simulink model "ref_submodel2"  (R2022b)
settings: Solver=FixedStepDiscrete  StartTime=0.0  StopTime=inf  RelTol=1e-3  EnableMultiTasking=on
libraries: speedgoatlib_IO135 x2, simulink x2, hdlsllib x2, slrealtimeloglib x1
settings Model: Creator=dmankov  LastModifiedBy=padlewsk
settings SolverCC: ConcurrentTasks=on  AlgebraicLoopSolver=TrustRegion  PositivePriorityOrder=on  AutoInsertRateTranBlk=on  InsertRTBMode=Never (minimum delay)
settings DataIOCC: SaveFormat=StructureWithTime
settings OptimizationCC: BlockReduction=off  OptimizeBlockIOStorage=off  BufferReuse=off  ReuseModelBlockBuffer=on  GlobalBufferReuse=off  ExpressionFolding=off  LocalBlockOutputs=off  OptimizeDataStoreBuffers=off  BusAssignmentInplaceUpdate=off
settings DebuggingCC: TasksWithSamePriorityMsg=none  UnconnectedInputMsg=warning  UnconnectedOutputMsg=warning  UnconnectedLineMsg=warning  ArithmeticOperatorsInVariantConditions=warning
settings HardwareCC: ProdBitPerLong=64  ProdLongLongMode=on  ProdHWDeviceType=Intel->x86-64 (Linux 64)
settings ModelReferenceCC: EnableRefExpFcnMdlSchedulingChecks=on  ModelReferenceNumInstancesAllowed=Single
settings SFSimCC: CustomCodeUndefinedFunction=UseInterfaceOnly
settings RTWCC: Description=Simulink Real-Time  SystemTargetFile=slrealtime.tlc  TemplateMakefile=slrealtime_default_tmf  Toolchain=Simulink Real-Time Toolchain  BuildConfiguration=Faster Runs  CodeExecutionProfiling=on  TargetLang=C++  DLArmComputeVersion=19.05
settings SimulinkRealTimeTargetCC: UseGCCFastMath=on

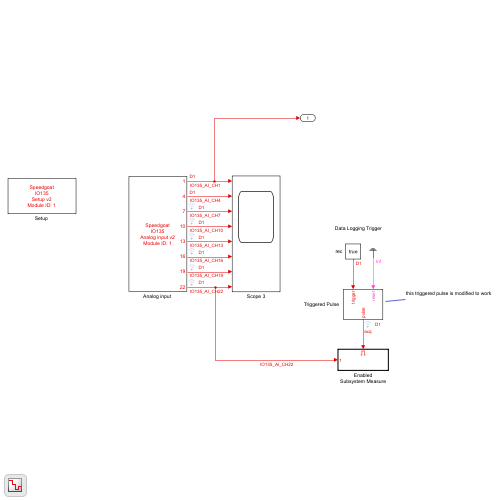
[thumbnail: Simulink's stored preview of the top-level diagram]
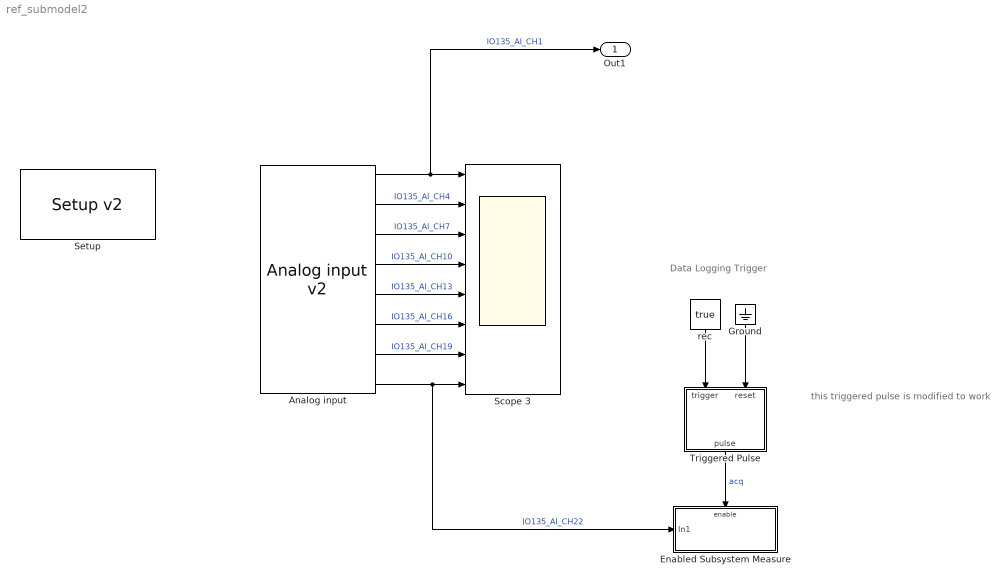
== system ref_submodel2 ==
  note: this triggered pulse is modified to work
  note: Data Logging Trigger
  "Analog input " : speedgoatlib_IO135/Analog input v2   parModuleId=1  parSampleTime=ts  parPciSlot=-1  parAdcChannels=[1 4 7 10 13 16 19 22]  parAdcVoltageRange=[2 2 2 2]  parAdcOversamplRate=[1 1 1 1]  parAdcContSampling=0  parAdcDmaEnable=0  parAdcActiveDmaDevices=[1 1 1 1]  parAdcFrameSize=50
      settings: SourceProductName=Simulink Real-Time: Speedgoat I/O Blockset
  Enabled Subsystem Measure : Subsystem  TreatAsAtomicUnit=on
  Ground : Ground
  Scope 3 : Scope  NumInputPorts=8
  "Setup " : speedgoatlib_IO135/Setup v2   parPciSlot=-1  parModuleId=1  parInterModuleSync=None  parConvClockBaseRate=20MHz  parConvClock1Divider=200  parConvClock2Divider=20000  parFrameTriggerEnable=off  parFrameTriggerDivider=10  parConvClock1BaseRate=1  parConvClock2BaseRate=1  parFrameTriggerClock=1  parAdcChannels=[1 4 7 10 13 16 19 22]  parAdcRange1=+-10V  parAdcRange2=+-10V  parAdcRange3=+-10V  parAdcRange4=+-10V  parAdcVoltageRange=[2 2 2 2]  parAdcOversampling1=None  parAdcOversampling2=None  parAdcOversampling3=None  parAdcOversampling4=None  parAdcOversamplRate=[1 1 1 1]  parAdcAutoCorrection=on  parAdcContSampling=off  parAdcDmaEnable=off  parAdcDmaClock=Clock 1  parAdcFrameSize_=50  parAdcSampleTime_=-1  parAdcActiveDmaDevices=[1 1 1 1]  parAdcFrameTriggerEnable=0  parAdcFrameSize=50  parAdcSampleTime=0.0005  parDacChannels=1:2:16  parDacInitValues=0  parDacReset=1  parDacRange1=+-10V  parDacRange2=+-10V  parDacRange3=+-10V  parDacRange4=+-10V  parDacRange5=+-10V  parDacRange6=+-10V  parDacRange7=+-10V  parDacRange8=+-10V  parDacRange9=+-10V  parDacRange10=+-10V  parDacRange11=+-10V  parDacRange12=+-10V  parDacRange13=+-10V  parDacRange14=+-10V  parDacRange15=+-10V  parDacRange16=+-10V  parDacVoltageRange=[5 5 5 5 5 5 5 5 5 5 5 5 5 5 5 5]  parDacAutoCorrection=on  parDacSyncOut=on  parDacDmaEnable=off  parDacDmaLatency=Until next frame  parDacDmaClock=Clock 1  parDacFrameSize_=100  parDacSampleTime_=-1  parDacActiveDmaDevices=[1 1 1 1]  parDacFrameTriggerEnable=0  parDacFrameSize=100  parDacSampleTime=0.001  parDoChannels=1:4  parDoInitValues=0  parDoReset=1  parDiChannels=5:8  parDiDebounceEnable=off  parDiDebounceTime=0  parDiDebounceValue=0  parDioPullRefFront=Pull-up 3.3V  parDioPullRefRear=Floating
      settings: SourceProductName=Simulink Real-Time: Speedgoat I/O Blockset
  "Triggered Pulse " : Subsystem  mask(Triggered Pulse){N=3000}
      mask prompts: N "Length (N samples)"
      mask help: Generates a single pulse of N samples length
  rec : Constant  Value=true  SampleTime=-1
  Out1 : Outport
  wires:
  "Analog input "/7 -> Scope 3/7  "IO135_AI_CH19"
  "Analog input "/8 -> Enabled Subsystem Measure/1(In1), Scope 3/8  "IO135_AI_CH22"
  "Analog input "/1 -> Out1/1, Scope 3/1  "IO135_AI_CH1"
  "Analog input "/3 -> Scope 3/3  "IO135_AI_CH7"
  "Analog input "/4 -> Scope 3/4  "IO135_AI_CH10"
  "Analog input "/6 -> Scope 3/6  "IO135_AI_CH16"
  "Analog input "/5 -> Scope 3/5  "IO135_AI_CH13"
  "Analog input "/2 -> Scope 3/2  "IO135_AI_CH4"
  "Triggered Pulse "/1(pulse) -> Enabled Subsystem Measure/Enable  "acq"
  rec/1 -> "Triggered Pulse "/1(trigger)
  Ground/1 -> "Triggered Pulse "/2(reset)

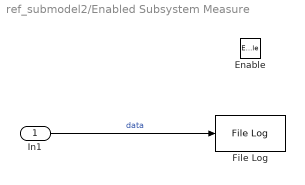
== system ref_submodel2/Enabled Subsystem Measure ==
  In1 : Inport
  Enable : EnablePort
  File Log : slrealtimeloglib/File Log  decimation=1  inputProcessing=Elements as channels (sample based)
  wires:
  In1/1 -> File Log/1  "data"

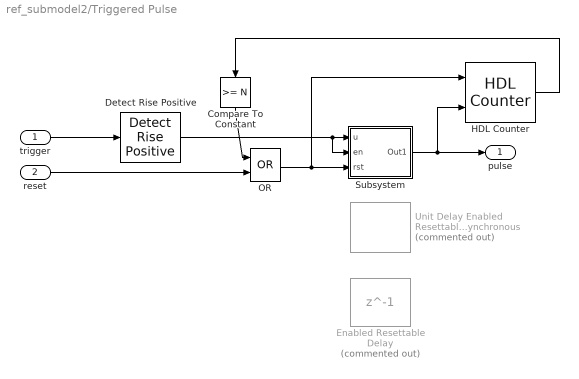
== system ref_submodel2/Triggered Pulse  ==
  trigger : Inport
  reset : Inport  Port=2
  Compare To Constant : simulink/Logic and Bit Operations/Compare To Constant  relop=>=  const=N  OutDataTypeStr=boolean
  Detect Rise Positive : simulink/Logic and Bit Operations/Detect Rise Positive  vinit=0  OutDataTypeStr=boolean
  Enabled Resettable Delay : Delay  Commented=on  DelayLength=1  ExternalReset=Level  ShowEnablePort=on
      settings: InputPortMap=u0,e6,r5
  HDL Counter : hdlsllib/Sources/HDL Counter  CountType=Free running  CountInit=1  CountStep=1  CountMax=25  CountFromType=Initial value  CountFrom=1  CountResetPort=on  CountLoadPort=off  CountEnbPort=on  CountDirPort=off  CountHitOutputPort=off  CountDataType=Unsigned  CountWordLen=32  CountFracLen=0  CountSampTime=1
  OR : Logic  Operator=OR  AllPortsSameDT=off  OutDataTypeStr=boolean
  Subsystem : Subsystem
  Unit Delay Enabled Resettable Synchronous : hdlsllib/Discrete/Unit Delay Enabled Resettable Synchronous  Commented=on  InitialCondition=0.0  SampleTime=-1
  pulse : Outport  VectorParamsAs1DForOutWhenUnconnected=off
  wires:
  OR/1 -> Subsystem/3(rst), HDL Counter/1
  trigger/1 -> Detect Rise Positive/1
  Subsystem/1(Out1) -> HDL Counter/2, pulse/1
  Compare To Constant/1 -> OR/1
  reset/1 -> OR/2
  Detect Rise Positive/1 -> Subsystem/2(en), Subsystem/1(u)
  HDL Counter/1 -> Compare To Constant/1

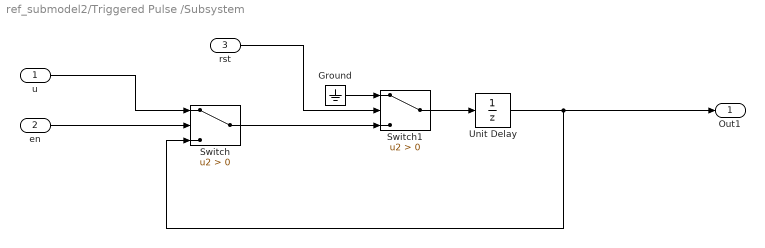
== system ref_submodel2/Triggered Pulse /Subsystem ==
  u : Inport
  en : Inport  Port=2
  rst : Inport  Port=3
  Ground : Ground
  Switch : Switch  Criteria=u2 > Threshold  SaturateOnIntegerOverflow=off  InputSameDT=off
  Switch1 : Switch  Criteria=u2 > Threshold  SaturateOnIntegerOverflow=off  InputSameDT=off
  Unit Delay : UnitDelay  SampleTime=-1  HasFrameUpgradeWarning=on
  Out1 : Outport
  wires:
  Unit Delay/1 -> Switch/3, Out1/1
  en/1 -> Switch/2
  u/1 -> Switch/1
  rst/1 -> Switch1/2
  Ground/1 -> Switch1/1
  Switch1/1 -> Unit Delay/1
  Switch/1 -> Switch1/3
